simulink model "simscapewithVisualization"  (R2021b)
settings: Solver=VariableStepAuto  StartTime=0.0  StopTime=10.0  RelTol=1e-3
values from neighbouring files (symbols this model uses):
  b = 0.1    [simscapeParameters.m]    (also in simscapeVisualization.m)
  R = 1    [simscapeParameters.m]    (also in simscapeVisualization.m)
libraries: fl_lib x10, nesl_utility x5, aerolibanimutils x1
settings Model: Creator=Joshua  LastModifiedBy=Joshua

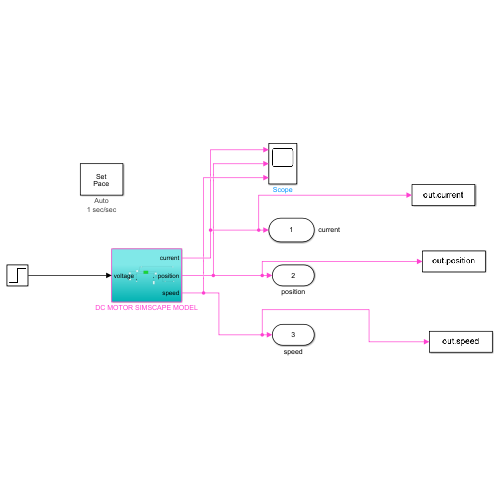
[thumbnail: Simulink's stored preview of the top-level diagram]
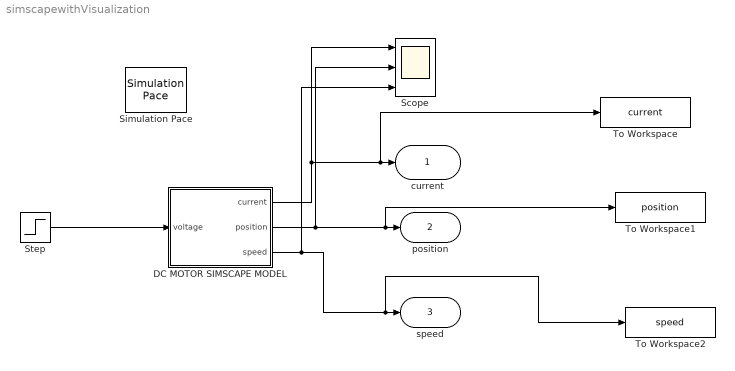
== system simscapewithVisualization ==
  DC MOTOR SIMSCAPE MODEL : Subsystem
  Scope : Scope  NumInputPorts=3
  Simulation Pace : aerolibanimutils/Simulation Pace  SimulationPace=1  SleepMode=Auto  OutputPaceError=off  SampleTime=1/30
  Step : Step  Time=0.1  After=12  SampleTime=0
  To Workspace : ToWorkspace  VariableName=current  SampleTime=-1
  To Workspace1 : ToWorkspace  VariableName=position  SampleTime=-1
  To Workspace2 : ToWorkspace  VariableName=speed  SampleTime=-1
  current : Outport
  position : Outport  Port=2
  speed : Outport  Port=3
  wires:
  DC MOTOR SIMSCAPE MODEL/2(position) -> Scope/2, To Workspace1/1, position/1
  Step/1 -> DC MOTOR SIMSCAPE MODEL/1(voltage)
  DC MOTOR SIMSCAPE MODEL/3(speed) -> Scope/3, To Workspace2/1, speed/1
  DC MOTOR SIMSCAPE MODEL/1(current) -> Scope/1, To Workspace/1, current/1

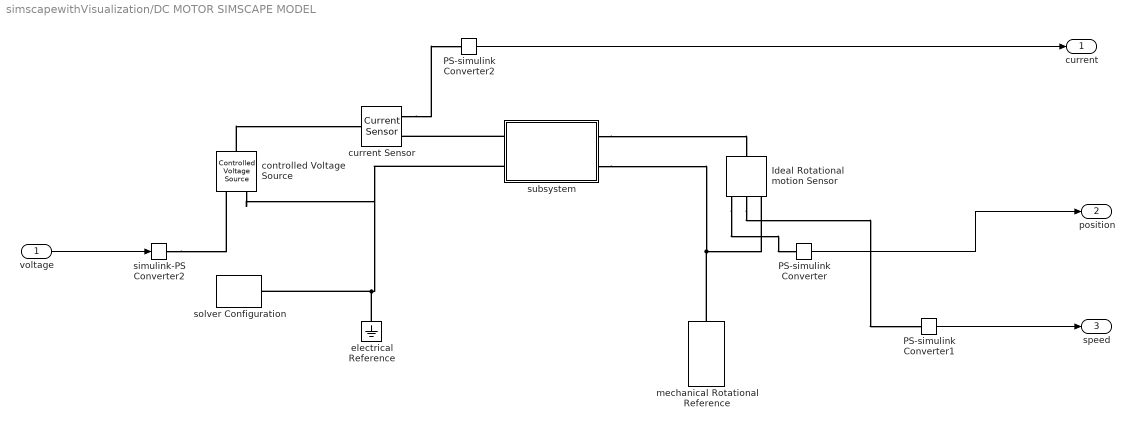
== system simscapewithVisualization/DC MOTOR SIMSCAPE MODEL ==
  voltage : Inport
  Ideal Rotational motion Sensor : fl_lib/Mechanical/Mechanical Sensors/Ideal Rotational Motion Sensor  wrap_angle=simscape.enum.onoff.off  offset=0 rad
  PS-simulink Converter : nesl_utility/PS-Simulink Converter  PhysicalDomain=network_engine_domain  SubClassName=ps_output  LeftPortType=input  RightPortType=output  PseudoPeriodic=off  Frequencies=[]  Unit=inherit  AffineConversion=off
      settings: SourceProductBaseCode=PW,SS
  PS-simulink Converter1 : nesl_utility/PS-Simulink Converter  PhysicalDomain=network_engine_domain  SubClassName=ps_output  LeftPortType=input  RightPortType=output  PseudoPeriodic=off  Frequencies=[]  Unit=inherit  AffineConversion=off
      settings: SourceProductBaseCode=PW,SS
  PS-simulink Converter2 : nesl_utility/PS-Simulink Converter  PhysicalDomain=network_engine_domain  SubClassName=ps_output  LeftPortType=input  RightPortType=output  PseudoPeriodic=off  Frequencies=[]  Unit=inherit  AffineConversion=off
      settings: SourceProductBaseCode=PW,SS
  controlled Voltage Source : fl_lib/Electrical/Electrical Sources/Controlled Voltage Source
  current Sensor : fl_lib/Electrical/Electrical Sensors/Current Sensor
  electrical Reference : fl_lib/Electrical/Electrical Elements/Electrical Reference
  mechanical Rotational Reference : fl_lib/Mechanical/Rotational Elements/Mechanical Rotational Reference
  simulink-PS Converter2 : nesl_utility/Simulink-PS Converter  PhysicalDomain=network_engine_domain  SubClassName=ps_input  LeftPortType=input  RightPortType=output  PseudoPeriodic=off  Frequencies=[]  NoiseDistribution=none  NoiseParameters=[]  Unit=1  AffineConversion=off  FilteringAndDerivatives=provide  SimscapeFilterOrder=1  InputFilterTimeConstant=0.001  UdotUserProvided=0
      settings: SourceProductBaseCode=PW,SS
  solver Configuration : nesl_utility/Solver Configuration  PhysicalDomain=network_engine_domain  SubClassName=solver  LeftPortType=input  RightPortType=generic  Tones=[]  Harmonics=[]  SimulateNoise=off  Profile=off  UseLocalSampling=off  EnableSwitchedLinearOptims=on  FrequencyDomain=off  UseCCode=off  RelTol=0.001  AbsTol=1e-06  MinStep=1e-09  ToWorkspace=off  RevertToSquareIcSolve=off  NumHomotopyIterations=100  PhasorMode=off  PhasorModeNumHarmonics=1  DoDC=off  ResidualTolerance=1e-09  UseLocalSolver=off  LocalSolverChoice=NE_BACKWARD_EULER_ADVANCER  LocalSolverSampleTime=0.001  DoFixedCost=off  MaxNonlinIter=3  MaxModeIter=2  ComputeImpulses=off  ImpulseIterations=2  LinearAlgebra=auto  EquationFormulation=NE_TIME_EF  DelaysMemoryBudget=1024  AutomaticFiltering=on  FilteringTimeConstant=0.001  PartitionStorageMethod=AS_NEEDED  PartitionMemoryBudget=1024  PartitionMethod=ROBUST
      settings: SourceProductBaseCode=PW,SS
  subsystem : Subsystem
  current : Outport
  position : Outport  Port=2
  speed : Outport  Port=3
  wires:
  PS-simulink Converter/1 -> position/1
  PS-simulink Converter2/1 -> current/1
  voltage/1 -> simulink-PS Converter2/1
  PS-simulink Converter1/1 -> speed/1
  connections:
  current Sensor/RConn1 -- PS-simulink Converter2/LConn1
  simulink-PS Converter2/RConn1 -- controlled Voltage Source/RConn1
  electrical Reference/LConn1 -- solver Configuration/RConn1 -- controlled Voltage Source/RConn2 -- subsystem/LConn2
  subsystem/RConn2 -- Ideal Rotational motion Sensor/RConn1 -- mechanical Rotational Reference/LConn1
  subsystem/RConn1 -- Ideal Rotational motion Sensor/LConn1
  controlled Voltage Source/LConn1 -- current Sensor/LConn1
  subsystem/LConn1 -- current Sensor/RConn2
  Ideal Rotational motion Sensor/RConn3 -- PS-simulink Converter/LConn1
  Ideal Rotational motion Sensor/RConn2 -- PS-simulink Converter1/LConn1

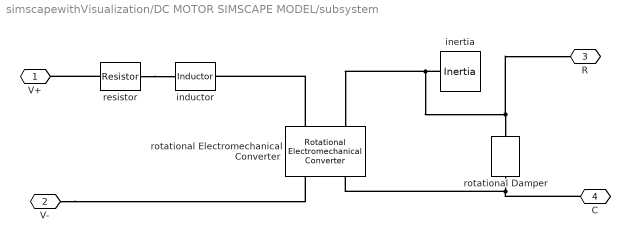
== system simscapewithVisualization/DC MOTOR SIMSCAPE MODEL/subsystem ==
  inductor : fl_lib/Electrical/Electrical Elements/Inductor  l=L H  r=0 Ohm  g=1e-9 1/Ohm  i_specify=off  i_priority=None  i=0 A  i_nominal_specify=off  i_nominal_unit=A  i_nominal_value=1  v_specify=off  v_priority=None  v=0 V  v_nominal_specify=off  v_nominal_unit=V  v_nominal_value=1  i_L_specify=off  i_L_priority=High  i_L=0 A  i_L_nominal_specify=off  i_L_nominal_unit=A  i_L_nominal_value=1
  inertia : fl_lib/Mechanical/Rotational Elements/Inertia  inertia=J kg*m^2  num_ports=foundation.enum.numPorts2.one  w_specify=off  w_priority=High  w=0 rad/s  w_nominal_specify=off  w_nominal_unit=rad/s  w_nominal_value=1  t_specify=off  t_priority=None  t=0 N*m  t_nominal_specify=off  t_nominal_unit=N*m  t_nominal_value=1
  resistor : fl_lib/Electrical/Electrical Elements/Resistor  R=R Ohm  i_specify=off  i_priority=None  i=0 A  i_nominal_specify=off  i_nominal_unit=A  i_nominal_value=1  v_specify=off  v_priority=None  v=0 V  v_nominal_specify=off  v_nominal_unit=V  v_nominal_value=1
  rotational Electromechanical Converter : fl_lib/Electrical/Electrical Elements/Rotational Electromechanical Converter  K=0.1 V*s/rad  i_specify=off  i_priority=None  i=0 A  i_nominal_specify=off  i_nominal_unit=A  i_nominal_value=1  v_specify=off  v_priority=None  v=0 V  v_nominal_specify=off  v_nominal_unit=V  v_nominal_value=1  t_specify=off  t_priority=None  t=0 N*m  t_nominal_specify=off  t_nominal_unit=N*m  t_nominal_value=1  w_specify=off  w_priority=None  w=0 rad/s  w_nominal_specify=off  w_nominal_unit=rad/s  w_nominal_value=1
  rotational Damper : fl_lib/Mechanical/Rotational Elements/Rotational Damper  D=b N*m/(rad/s)  w_specify=off  w_priority=None  w=0 rad/s  w_nominal_specify=off  w_nominal_unit=rad/s  w_nominal_value=1  t_specify=off  t_priority=None  t=0 N*m  t_nominal_specify=off  t_nominal_unit=N*m  t_nominal_value=1
  V+ : PMIOPort  Side=Left
  V- : PMIOPort  Port=2  Side=Left
  R : PMIOPort  Port=3  Side=Right
  C : PMIOPort  Port=4  Side=Right
  connections:
  V-/RConn1 -- rotational Electromechanical Converter/RConn1
  inertia/LConn1 -- rotational Electromechanical Converter/LConn2 -- rotational Damper/RConn1 -- R/RConn1
  rotational Damper/LConn1 -- rotational Electromechanical Converter/RConn2 -- C/RConn1
  resistor/LConn1 -- V+/RConn1
  resistor/RConn1 -- inductor/LConn1
  rotational Electromechanical Converter/LConn1 -- inductor/RConn1
